simulink model "lookup_table"  (R2020b)
settings: Solver=VariableStepAuto  StartTime=0.0  StopTime=10.0  RelTol=1e-3
values from neighbouring files (symbols this model uses):
  fwd_bias_v = [0 0.1 0.2 0.3 0.4 0.6 0.8 1.0 1.2 1.4 1.6 1.8 2.0 2.2 2.4]    [initial_values.m]
  fwd_current = [0 0 0 0 0.5 1 2 3 5 7.5 10 15 20 25 30]    [initial_values.m]
  reverse_bias_v = [0 5 7 9 11 13 15 17 19 21 23 25]    [initial_values.m]
  reverse_current = [0 1 2 3 4 5 7 9 11 13 15 25]    [initial_values.m]
libraries: dspsrcs4 x2
settings Model: Creator=shubham sharma  LastModifiedBy=shubham sharma

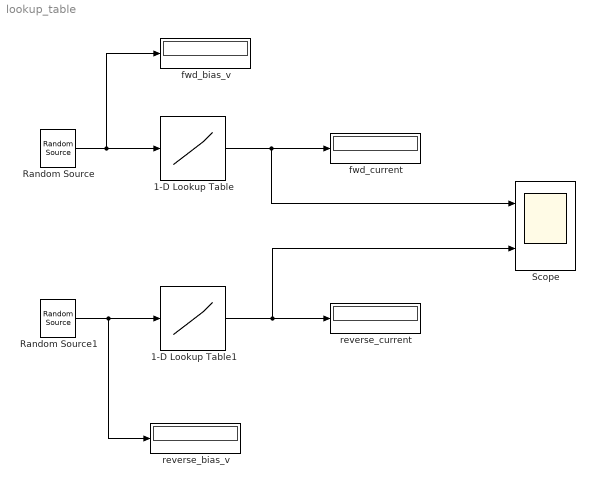
== system lookup_table ==
  1-D Lookup Table : Lookup_n-D  NumberOfTableDimensions=1  BreakpointsForDimension1=fwd_bias_v  Table=fwd_current  InternalRulePriority=Speed  RndMeth=Simplest  InputSameDT=on
  1-D Lookup Table1 : Lookup_n-D  NumberOfTableDimensions=1  BreakpointsForDimension1=reverse_bias_v  Table=reverse_current  InternalRulePriority=Speed  RndMeth=Simplest  InputSameDT=on
  Random Source : dspsrcs4/Random Source  SrcType=Uniform  NormMethod=Ziggurat  CltLength=12  MinVal=0  MaxVal=2.4  MeanVal=0  VarVal=1  RepMode=Not repeatable  rawSeed=1  IsInherit=off  SampMode=Discrete  SampTime=1  SampFrame=1  DataType=Double  OutComplex=Real  OutputFrames=off
  Random Source1 : dspsrcs4/Random Source  SrcType=Uniform  NormMethod=Ziggurat  CltLength=12  MinVal=0  MaxVal=25  MeanVal=0  VarVal=1  RepMode=Not repeatable  rawSeed=1  IsInherit=off  SampMode=Discrete  SampTime=1  SampFrame=1  DataType=Double  OutComplex=Real  OutputFrames=off
  Scope : Scope  NumInputPorts=2
  fwd_bias_v : Display
  fwd_current : Display
  reverse_bias_v : Display
  reverse_current : Display
  wires:
  Random Source/1 -> fwd_bias_v/1, 1-D Lookup Table/1
  1-D Lookup Table/1 -> Scope/1, fwd_current/1
  Random Source1/1 -> reverse_bias_v/1, 1-D Lookup Table1/1
  1-D Lookup Table1/1 -> Scope/2, reverse_current/1
